simulink model "lkaLaneTrackingMdl_SFcn_test"  (Simulink 7.9)
settings: Solver=ode45  StartTime=0.0  StopTime=10.0  RelTol=1e-3
settings Model: Creator=georgnestlinger  LastModifiedBy=georgnestlinger
settings DebuggingCC: SolverPrmCheckMsg=none

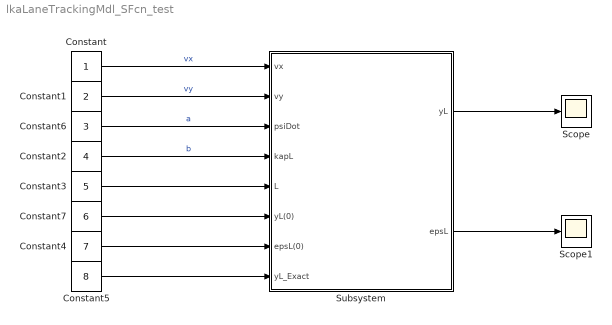
== system lkaLaneTrackingMdl_SFcn_test ==
  Constant : Constant
  Constant1 : Constant  Value=2
  Constant2 : Constant  Value=4
  Constant3 : Constant  Value=5
  Constant4 : Constant  Value=7
  Constant5 : Constant  Value=8
  Constant6 : Constant  Value=3
  Constant7 : Constant  Value=6
  Scope : Scope
  Scope1 : Scope
  Subsystem : Subsystem
  wires:
  Constant/1 -> Subsystem/1(vx)  "vx"
  Subsystem/1(yL) -> Scope/1
  Constant1/1 -> Subsystem/2(vy)  "vy"
  Constant6/1 -> Subsystem/3(psiDot)  "a"
  Constant3/1 -> Subsystem/5(L)
  Subsystem/2(epsL) -> Scope1/1
  Constant4/1 -> Subsystem/7(epsL(0))
  Constant2/1 -> Subsystem/4(kapL)  "b"
  Constant7/1 -> Subsystem/6(yL(0))
  Constant5/1 -> Subsystem/8(yL_Exact)

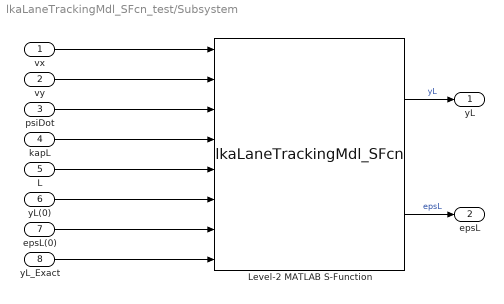
== system lkaLaneTrackingMdl_SFcn_test/Subsystem ==
  vx : Inport
  vy : Inport  Port=2
  psiDot : Inport  Port=3
  kapL : Inport  Port=4
  L : Inport  Port=5
  yL(0) : Inport  Port=6
  epsL(0) : Inport  Port=7
  yL_Exact : Inport  Port=8
  Level-2 MATLAB S-Function : M-S-Function  FunctionName=lkaLaneTrackingMdl_SFcn
  yL : Outport
  epsL : Outport  Port=2
  wires:
  vx/1 -> Level-2 MATLAB S-Function/1
  vy/1 -> Level-2 MATLAB S-Function/2
  Level-2 MATLAB S-Function/1 -> yL/1  "yL"
  psiDot/1 -> Level-2 MATLAB S-Function/3
  kapL/1 -> Level-2 MATLAB S-Function/4
  L/1 -> Level-2 MATLAB S-Function/5
  Level-2 MATLAB S-Function/2 -> epsL/1  "epsL"
  yL(0)/1 -> Level-2 MATLAB S-Function/6
  epsL(0)/1 -> Level-2 MATLAB S-Function/7
  yL_Exact/1 -> Level-2 MATLAB S-Function/8
